simulink model "SpatialKineticsOffline"  (R2013a)
settings: Solver=ode4  StartTime=0.0  StopTime=tf  FixedStep=.001  RelTol=1e-3
PreLoadFcn:
  | load DarkLowerCoeffs
  | load DarkMiddleCoeffs
  | load DarkUpperCoeffs
  | load breaks
values from neighbouring files (symbols this model uses):
  alpha = [ -2.61*pcm -0.53*pcm ]    [SpatialKineticsOpenSourceMain.m]
  breaks = DarkLowerBreaks    [SpatialKineticsOpenSourceMain.m]
  BRIO = 4.266e7    (= 42660000)    [SpatialKineticsOpenSourceMain.m]
  cpc = 2414    [SpatialKineticsOpenSourceMain.m]
  cpp = 2414    [SpatialKineticsOpenSourceMain.m]
  DarkLowerCoeffs = ppDarkLower.coefs    [SpatialKineticsOpenSourceMain.m]
  DarkMiddleCoeffs = ppDarkMiddle.coefs    [SpatialKineticsOpenSourceMain.m]
  DarkRodWorthInserted = -5*Beta    (= -0.00815)    [SpatialKineticsOpenSourceMain.m]
  DarkUpperCoeffs = ppDarkUpper.coefs    [SpatialKineticsOpenSourceMain.m]
  downcomerTimeConstant = 5    [SpatialKineticsOpenSourceMain.m]
  downIO = 216.6*ones(1,3)    [SpatialKineticsOpenSourceMain.m]
  Kc1 = 1/(rho_secondary*V_secondary)    (= 0.00032726218348)    [SpatialKineticsOpenSourceMain.m]
  Kc2 = (h_secondary*A)/(cps*rho_secondary*V_secondary)    (= 1.23242359038)    [SpatialKineticsOpenSourceMain.m]
  Kh1 = 1/(rho_primary*V_primary)    (= 0.000447917898441)    [SpatialKineticsOpenSourceMain.m]
  Kh2 = (h_primary*A)/(cpp*rho_primary*V_primary)    (= 1.29038206968)    [SpatialKineticsOpenSourceMain.m]
  Kw1 = h_primary    (= 23800)    [SpatialKineticsOpenSourceMain.m]
  Kw2 = h_secondary    (= 24500)    [SpatialKineticsOpenSourceMain.m]
  Kw3 = A/(rho_tube*cpw*V_tube)    (= 0.000122049789882)    [SpatialKineticsOpenSourceMain.m]
  PHX_IO = [649.8 637.9 643.7]    [SpatialKineticsOpenSourceMain.m]
  PHX_PI_IO = 271.8    [SpatialKineticsOpenSourceMain.m]
  rate_pct = rate/100    [SpatialKineticsOfflineMain.m]
  rcp_activatetime = 20    [SpatialKineticsOpenSourceMain.m]
  rcpt = 0.1    [SpatialKineticsOpenSourceMain.m]
  reactor_PI_IO = 0.8574    [SpatialKineticsOpenSourceMain.m]
  SVIO = zeros(1,17)    [SpatialKineticsOpenSourceMain.m]
  Ts = 0.001    [SpatialKineticsOpenSourceMain.m]
  xfc0 = -Atemp\btemp*u0    [SpatialKineticsOpenSourceMain.m]
  zone1_IO = [1.041 0.01764 0.04848]    [SpatialKineticsOpenSourceMain.m]
  zone1_thermal_IO = [1044 658.3]    [SpatialKineticsOpenSourceMain.m]
  zone2_IO = [1.098 0.0186 0.05114]    [SpatialKineticsOpenSourceMain.m]
  zone2_thermal_IO = [1083 675.9]    [SpatialKineticsOpenSourceMain.m]
  zone3_IO = [0.9147 0.01549 0.04259]    [SpatialKineticsOpenSourceMain.m]
  zone3_thermal_IO = [1031 692.5]    [SpatialKineticsOpenSourceMain.m]
libraries: simulink x36
(part 4 of 5)

== system SpatialKineticsOffline/RX #3/Primary Heat Exchanger Lumped Model #5 ==
  Primary mass flow  in : Inport
  Primary temp in : Inport  Port=2
  Secondary temp in : Inport  Port=3
  Secondary mass flow in : Inport  Port=4
  Constant : Constant  Value=Kh1  SampleTime=Ts
  Constant1 : Constant  Value=Kh2  SampleTime=Ts
  Constant2 : Constant  Value=Kc1  SampleTime=Ts
  Constant3 : Constant  Value=Kc2  SampleTime=Ts
  Constant4 : Constant  Value=Kw1  SampleTime=Ts
  Constant5 : Constant  Value=Kw2  SampleTime=Ts
  Constant6 : Constant  Value=Kw3  SampleTime=Ts
  Constant7 : Constant  Value=cpp  SampleTime=Ts
  Demux : Demux  Outputs=3
  Display : Display
  Integrator : Integrator  InitialCondition=PHX_IO
  MATLAB Function : MATLAB Function  TreatAsAtomicUnit=on
  Mux2 : Mux  Inputs=7
  Product : Product
  Product1 : Product
  Sum : Sum  Inputs=|+-
  Terminator : Terminator
  W to MW : Gain  Gain=1e-6
  PHx1_Tho : Outport
  PHx1_Tco : Outport  Port=2
  PHx1_HXout : Outport  Port=3
  wires:
  Constant/1 -> Mux2/1
  Constant1/1 -> Mux2/2
  Constant2/1 -> Mux2/3
  Constant3/1 -> Mux2/4
  Constant4/1 -> Mux2/5
  Constant5/1 -> Mux2/6
  Constant6/1 -> Mux2/7
  Mux2/1 -> [PHXpar]
  MATLAB Function/1(dx) -> Integrator/1
  [PHXpar] -> MATLAB Function/6(hxpar)
  Primary temp in/1 -> [Thi], MATLAB Function/2(Thi_input)
  Secondary temp in/1 -> MATLAB Function/3(Tci_input)
  Secondary mass flow in/1 -> MATLAB Function/5(mdotc_input)
  Primary mass flow  in/1 -> [mdoth], MATLAB Function/4(mdoth_input)
  Demux/3 -> Terminator/1
  Demux/2 -> PHx1_Tco/1
  Demux/1 -> [Tho], PHx1_Tho/1
  Constant7/1 -> Product/2
  [mdoth] -> Product/1
  [Thi] -> Sum/1
  [Tho] -> Sum/2
  Product/1 -> Product1/1
  Sum/1 -> Product1/2
  Product1/1 -> W to MW/1
  W to MW/1 -> PHx1_HXout/1
  Integrator/1 -> Display/1, MATLAB Function/1(x), Demux/1

== system SpatialKineticsOffline/RX #3/Primary Heat Exchanger Lumped Model #6 ==
  Primary mass flow  in : Inport
  Primary temp in : Inport  Port=2
  Secondary temp in : Inport  Port=3
  Secondary mass flow in : Inport  Port=4
  Constant : Constant  Value=Kh1  SampleTime=Ts
  Constant1 : Constant  Value=Kh2  SampleTime=Ts
  Constant2 : Constant  Value=Kc1  SampleTime=Ts
  Constant3 : Constant  Value=Kc2  SampleTime=Ts
  Constant4 : Constant  Value=Kw1  SampleTime=Ts
  Constant5 : Constant  Value=Kw2  SampleTime=Ts
  Constant6 : Constant  Value=Kw3  SampleTime=Ts
  Constant7 : Constant  Value=cpp  SampleTime=Ts
  Demux : Demux  Outputs=3
  Display : Display
  Integrator : Integrator  InitialCondition=PHX_IO
  MATLAB Function : MATLAB Function  TreatAsAtomicUnit=on
  Mux2 : Mux  Inputs=7
  Product : Product
  Product1 : Product
  Sum : Sum  Inputs=|+-
  Terminator : Terminator
  W to MW : Gain  Gain=1e-6
  PHx1_Tho : Outport
  PHx1_Tco : Outport  Port=2
  PHx1_HXout : Outport  Port=3
  wires:
  Constant/1 -> Mux2/1
  Constant1/1 -> Mux2/2
  Constant2/1 -> Mux2/3
  Constant3/1 -> Mux2/4
  Constant4/1 -> Mux2/5
  Constant5/1 -> Mux2/6
  Constant6/1 -> Mux2/7
  Mux2/1 -> [PHXpar]
  MATLAB Function/1(dx) -> Integrator/1
  [PHXpar] -> MATLAB Function/6(hxpar)
  Primary temp in/1 -> [Thi], MATLAB Function/2(Thi_input)
  Secondary temp in/1 -> MATLAB Function/3(Tci_input)
  Secondary mass flow in/1 -> MATLAB Function/5(mdotc_input)
  Primary mass flow  in/1 -> [mdoth], MATLAB Function/4(mdoth_input)
  Integrator/1 -> Display/1, Demux/1, MATLAB Function/1(x)
  Demux/3 -> Terminator/1
  Demux/2 -> PHx1_Tco/1
  Demux/1 -> [Tho], PHx1_Tho/1
  Constant7/1 -> Product/2
  [mdoth] -> Product/1
  [Thi] -> Sum/1
  [Tho] -> Sum/2
  Product/1 -> Product1/1
  Sum/1 -> Product1/2
  Product1/1 -> W to MW/1
  W to MW/1 -> PHx1_HXout/1

== system SpatialKineticsOffline/RX #3/Ramp Power1 ==
  Max Demand : Inport
  Add : Sum
  Clock : Clock
  Ramp : simulink/Sources/Ramp  slope=rate_pct*42/60  start=tf/2  X0=-rate_pct*42/60*tf/2
  Ramp1 : simulink/Sources/Ramp  slope=-rate_pct*42/60  start=0  X0=0
  Switch : Switch  Threshold=tf/2
  Current Demand : Outport
  wires:
  Switch/1 -> Add/2
  Clock/1 -> Switch/2
  Ramp1/1 -> Switch/3
  Ramp/1 -> Switch/1
  Add/1 -> Current Demand/1
  Max Demand/1 -> Add/1

== system SpatialKineticsOffline/RX #3/Ramp Power2 ==
  Max Demand : Inport
  Add : Sum
  Clock : Clock
  Ramp : simulink/Sources/Ramp  slope=rate_pct*42/60  start=tf/2  X0=-rate_pct*42/60*tf/2
  Ramp1 : simulink/Sources/Ramp  slope=-rate_pct*42/60  start=0  X0=0
  Switch : Switch  Threshold=tf/2
  Current Demand : Outport
  wires:
  Switch/1 -> Add/2
  Clock/1 -> Switch/2
  Ramp1/1 -> Switch/3
  Ramp/1 -> Switch/1
  Add/1 -> Current Demand/1
  Max Demand/1 -> Add/1

== system SpatialKineticsOffline/RX #3/Ramp Power3 ==
  Max Demand : Inport
  Add : Sum
  Clock : Clock
  Ramp : simulink/Sources/Ramp  slope=rate_pct*42/60  start=tf/2  X0=-rate_pct*42/60*tf/2
  Ramp1 : simulink/Sources/Ramp  slope=-rate_pct*42/60  start=0  X0=0
  Switch : Switch  Threshold=tf/2
  Current Demand : Outport
  wires:
  Switch/1 -> Add/2
  Clock/1 -> Switch/2
  Ramp1/1 -> Switch/3
  Ramp/1 -> Switch/1
  Add/1 -> Current Demand/1
  Max Demand/1 -> Add/1

== system SpatialKineticsOffline/RX #3/Reactor Outlet Temperature PI Controller1 ==
  In1 : Inport
  Display : Display
  Display1 : Display
  Display2 : Display
  Gain2 : Gain  Gain=0.01
  Gain5 : Gain  Gain=100
  Integrator : Integrator  InitialCondition=reactor_PI_IO
  Kp : Gain  Gain=.01
  Saturation : Saturate  UpperLimit=1  LowerLimit=0
  Sum12 : Sum  Inputs=+-|
  Sum13 : Sum  Inputs=|+-
  Sum2 : Sum  Inputs=|++
  Out1 : Outport
  wires:
  In1/1 -> Kp/1, Sum13/1
  Sum2/1 -> Display/1, Sum12/1, Saturation/1
  Gain2/1 -> Integrator/1
  Integrator/1 -> Display2/1, Sum2/2
  Kp/1 -> Display1/1, Sum2/1
  Saturation/1 -> Sum12/2, Out1/1
  Sum12/1 -> Gain5/1
  Sum13/1 -> Gain2/1
  Gain5/1 -> Sum13/2

== system SpatialKineticsOffline/RX #3/Secondary-side RCP Dynamics #4 ==
  In1 : Inport
  Digital Clock #1 : DigitalClock  SampleTime=Ts
  RCP #1 : TransferFcn  Numerator=[rcpt]  Denominator=[1 rcpt]
  RCP Dynamics Switch #1 : Switch  Threshold=rcp_activatetime
  Out1 : Outport
  wires:
  In1/1 -> RCP #1/1, RCP Dynamics Switch #1/3
  Digital Clock #1/1 -> RCP Dynamics Switch #1/2
  RCP #1/1 -> RCP Dynamics Switch #1/1
  RCP Dynamics Switch #1/1 -> Out1/1

== system SpatialKineticsOffline/RX #3/Secondary-side RCP Dynamics #5 ==
  In1 : Inport
  Digital Clock#2 : DigitalClock  SampleTime=Ts
  RCP #2 : TransferFcn  Numerator=[rcpt]  Denominator=[1 rcpt]
  RCP Dynamics Switch #2 : Switch  Threshold=rcp_activatetime
  Out1 : Outport
  wires:
  RCP Dynamics Switch #2/1 -> Out1/1
  In1/1 -> RCP #2/1, RCP Dynamics Switch #2/3
  Digital Clock#2/1 -> RCP Dynamics Switch #2/2
  RCP #2/1 -> RCP Dynamics Switch #2/1

== system SpatialKineticsOffline/RX #3/Secondary-side RCP Dynamics #6 ==
  In1 : Inport
  Digital Clock #3 : DigitalClock  SampleTime=Ts
  RCP #3 : TransferFcn  Numerator=[rcpt]  Denominator=[1 rcpt]
  RCP Dynamics Switch #3 : Switch  Threshold=rcp_activatetime
  Out1 : Outport
  wires:
  RCP #3/1 -> RCP Dynamics Switch #3/1
  Digital Clock #3/1 -> RCP Dynamics Switch #3/2
  In1/1 -> RCP #3/1, RCP Dynamics Switch #3/3
  RCP Dynamics Switch #3/1 -> Out1/1

== system SpatialKineticsOffline/RX #4/Downcomer mixing dynamics ==
  PHX Primary Flow 1 : Inport
  PHX Primary Flow 2 : Inport  Port=2
  PHX Primary Flow 3 : Inport  Port=3
  PHX Primary Temp 1 : Inport  Port=4
  PHX Primary Temp 2 : Inport  Port=5
  PHX Primary Temp 3 : Inport  Port=6
  Constant5 : Constant  Value=[0,downcomerTimeConstant]
  Display : Display
  Integrator : Integrator  InitialCondition=downIO
  MATLAB Function1 : MATLAB Function  TreatAsAtomicUnit=on
  Primary Mass Flow Rate : Outport
  Temperature to Reactor T-H : Outport  Port=2
  wires:
  PHX Primary Flow 1/1 -> MATLAB Function1/1(m1)
  PHX Primary Flow 2/1 -> MATLAB Function1/2(m2)
  PHX Primary Flow 3/1 -> MATLAB Function1/3(m3)
  PHX Primary Temp 1/1 -> MATLAB Function1/4(t1)
  PHX Primary Temp 2/1 -> MATLAB Function1/5(t2)
  PHX Primary Temp 3/1 -> MATLAB Function1/6(t3)
  MATLAB Function1/3(xdot) -> Integrator/1
  Integrator/1 -> MATLAB Function1/8(x), Display/1
  MATLAB Function1/1(y) -> Temperature to Reactor T-H/1
  Constant5/1 -> MATLAB Function1/7(constants)
  MATLAB Function1/2(mtotal) -> Primary Mass Flow Rate/1

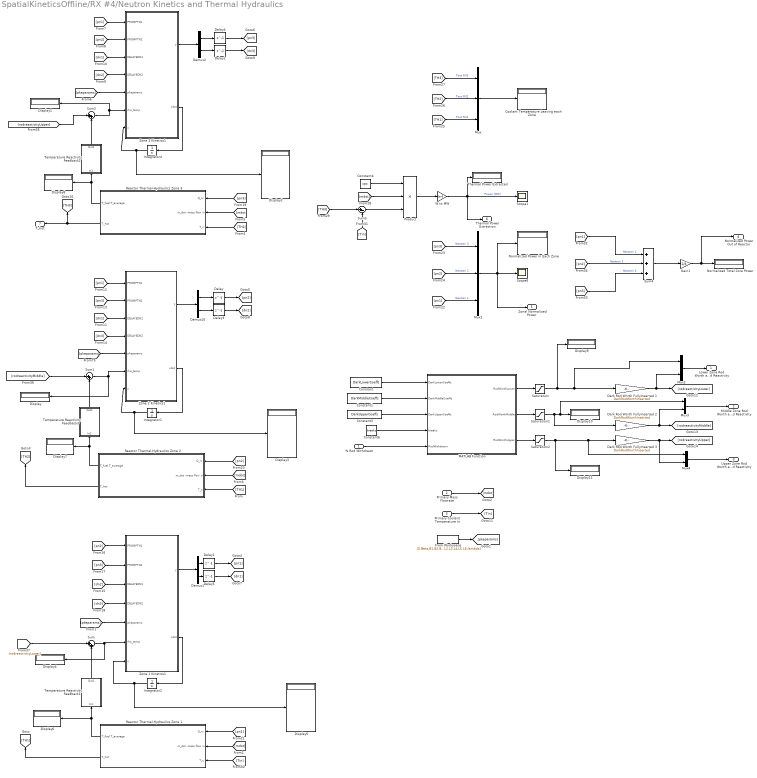
== system SpatialKineticsOffline/RX #4/Neutron Kinetics and Thermal Hydraulics ==
  % Rod Withdrawn : Inport
  Primary Mass Flowrate : Inport  Port=2
  Primary Coolant Temperature In : Inport  Port=3
  Constant : Constant  Value=DarkLowerCoeffs
  Constant1 : Constant  Value=DarkMiddleCoeffs
  Constant3 : Constant  Value=DarkUpperCoeffs
  Constant4 : Constant  Value=cpc
  Constant6 : Constant  Value=breaks
  Coolant Temperature Leaving each Zone : Display
  Dark Rod Worth FullyInserted 1 : Gain  Gain=DarkRodWorthInserted
  Dark Rod Worth FullyInserted 2 : Gain  Gain=DarkRodWorthInserted
  Dark Rod Worth FullyInserted 3 : Gain  Gain=DarkRodWorthInserted
  Delay{,1..5} (6 alike) : Delay  DelayLength=1  InitialCondition=0
  Demux1 : Demux  Outputs=2
  Demux10 : Demux  Outputs=2
  Demux2 : Demux  Outputs=2
  Display{,1..11} (12 alike) : Display
  From Workspace : FromWorkspace  VariableName=[0,Beta,B1,B2,B3,B4,B5,B6,L1,L2,L3,L4,L5,L6,lambda]  SampleTime=0
  Gain1 : Gain  Gain=1/3
  Integrator1 : Integrator  InitialCondition=zone2_IO
  Integrator2 : Integrator  InitialCondition=zone1_IO
  Integrator4 : Integrator  InitialCondition=zone3_IO
  MATLAB Function : MATLAB Function  TreatAsAtomicUnit=on
  Mux : Mux  Inputs=3
  Mux1 : Mux  Inputs=3
  Mux2 : Mux  Inputs=2
  Mux3 : Mux  Inputs=2
  Mux4 : Mux  Inputs=2
  Normalized Power in Each Zone : Display
  Normalized Total Core Power : Display
  Product : Product  Inputs=3
  Reactor Thermal-Hydraulics Zone 1 : Subsystem
  Reactor Thermal-Hydraulics Zone 2 : Subsystem
  Reactor Thermal-Hydraulics Zone 3 : Subsystem
  Saturation : Saturate  UpperLimit=inf  LowerLimit=0
  Saturation1 : Saturate  UpperLimit=inf  LowerLimit=0
  Saturation2 : Saturate  UpperLimit=inf  LowerLimit=0
  Scope1 : Scope
      settings: SaveName=ScopeData17
  Scope6 : Scope
      settings: SaveName=ScopeData16
  Sum : Sum  Inputs=|++
  Sum1 : Sum  Inputs=|++
  Sum2 : Sum  Inputs=|++
  Sum3 : Sum  Inputs=|+-
  Sum4 : Sum  Inputs=+++
  Temperature Reactivity Feedback1 : Subsystem
  Temperature Reactivity Feedback2 : Subsystem
  Temperature Reactivity Feedback3 : Subsystem
  Thermal Power Extracted : Display
  W to MW : Gain  Gain=1e-6
  Zone 1 Kinetics1 : MATLAB Function  TreatAsAtomicUnit=on
  Zone 2 Kinetics1 : MATLAB Function  TreatAsAtomicUnit=on
  Zone 3 Kinetics1 : MATLAB Function  TreatAsAtomicUnit=on
  Lower Zone Rod Worth and Reactivity : Outport
  Middle Zone Rod Worth and Reactivity : Outport  Port=2
  Upper Zone Rod Worth and Reactivity : Outport  Port=3
  Normalized Power Out of Reactor : Outport  Port=4
  Zonal Normalized Power : Outport  Port=5
  Thermal Power Extraction : Outport  Port=6
  T_hot : Outport  Port=7
  wires:
  [pkeparams] -> Zone 2 Kinetics1/5(pkeparams)
  Demux1/2 -> Delay5/1
  From Workspace/1 -> [pkeparams]
  Reactor Thermal-Hydraulics Zone 2/1(T_fuel,T_average) -> Display7/1, Temperature Reactivity Feedback3/1(In1)
  [TH1] -> Reactor Thermal-Hydraulics Zone 2/3(T_c)
  Temperature Reactivity Feedback3/1(Out1) -> Sum1/2
  [pkeparams] -> Zone 1 Kinetics1/5(pkeparams)
  Zone 1 Kinetics1/1(y) -> Demux1/1
  Reactor Thermal-Hydraulics Zone 1/1(T_fuel,T_average) -> Temperature Reactivity Feedback1/1(In1), Display6/1
  Temperature Reactivity Feedback1/1(Out1) -> Sum/2
  Demux1/1 -> Delay1/1
  Sum/1 -> Zone 1 Kinetics1/6(rho_temp), Display4/1
  [rodreactivityLower] -> Sum/1
  Sum1/1 -> Zone 2 Kinetics1/6(rho_temp), Display/1
  [rodreactivityMiddle] -> Sum1/1
  Mux/1 -> Coolant Temperature Leaving each Zone/1
  Reactor Thermal-Hydraulics Zone 1/2(T_hot) -> [TH1]
  [mdot] -> Reactor Thermal-Hydraulics Zone 2/2(m_dot -mass flow in)
  [mdot] -> Reactor Thermal-Hydraulics Zone 1/2(m_dot -mass flow in)
  Reactor Thermal-Hydraulics Zone 3/1(T_fuel,T_average) -> Display8/1, Temperature Reactivity Feedback2/1(In1)
  [TH2] -> Reactor Thermal-Hydraulics Zone 3/3(T_c)
  Reactor Thermal-Hydraulics Zone 3/2(T_hot) -> T_hot/1, [TH3]
  Temperature Reactivity Feedback2/1(Out1) -> Sum2/2
  Demux2/1 -> Delay4/1
  Sum2/1 -> Zone 3 Kinetics1/6(rho_temp), Display1/1
  [mdot] -> Reactor Thermal-Hydraulics Zone 3/2(m_dot -mass flow in)
  Delay5/1 -> [dn1]
  Demux2/2 -> Delay2/1
  Reactor Thermal-Hydraulics Zone 2/2(T_hot) -> [TH2]
  Demux10/1 -> Delay/1
  Demux10/2 -> Delay3/1
  Delay4/1 -> [pn3]
  Delay/1 -> [pn2]
  Delay1/1 -> [pn1]
  Delay3/1 -> [dn2]
  Delay2/1 -> [dn3]
  [rodreactivityUpper] -> Sum2/1
  [pn1] -> Zone 2 Kinetics1/1(PROMPTN1)
  [pn3] -> Zone 2 Kinetics1/2(PROMPTN2)
  [dn3] -> Zone 2 Kinetics1/4(DELAYEDN2)
  [dn1] -> Zone 2 Kinetics1/3(DELAYEDN1)
  [pn2] -> Zone 1 Kinetics1/1(PROMPTN1)
  [pn3] -> Zone 1 Kinetics1/2(PROMPTN2)
  [dn2] -> Zone 1 Kinetics1/3(DELAYEDN1)
  [dn3] -> Zone 1 Kinetics1/4(DELAYEDN2)
  [pn3] -> Reactor Thermal-Hydraulics Zone 3/1(Q_rx)
  [pn2] -> Reactor Thermal-Hydraulics Zone 2/1(Q_rx)
  [pn1] -> Reactor Thermal-Hydraulics Zone 1/1(Q_rx)
  Mux1/1 -> Scope6/1, Zonal Normalized Power/1, Normalized Power in Each Zone/1
  [pn1] -> Mux1/3  "Neutron 1"
  [pn3] -> Mux1/1  "Neutron 3"
  [pn2] -> Mux1/2  "Neutron 2"
  [TH1] -> Mux/3  "Tout RX1"
  [TH2] -> Mux/2  "Tout RX2"
  [TH3] -> Mux/1  "Tout RX3"
  Constant4/1 -> Product/1
  [mdot] -> Product/2
  Sum3/1 -> Product/3
  [TH3] -> Sum3/1
  [Tin] -> Reactor Thermal-Hydraulics Zone 1/3(T_c)
  [Tin] -> Sum3/2
  Product/1 -> W to MW/1
  W to MW/1 -> Scope1/1, Thermal Power Extraction/1, Thermal Power Extracted/1  "Power (MW)"
  [pn1] -> Sum4/1  "Neutron 1"
  [pn3] -> Sum4/3  "Neutron 3"
  [pn2] -> Sum4/2  "Neutron 2"
  Sum4/1 -> Gain1/1
  Gain1/1 -> Normalized Power Out of Reactor/1, Normalized Total Core Power/1
  Constant6/1 -> MATLAB Function/4(breaks)
  Constant3/1 -> MATLAB Function/3(DarkUpperCoeffs)
  Constant1/1 -> MATLAB Function/2(DarkMiddleCoeffs)
  Constant/1 -> MATLAB Function/1(DarkLowerCoeffs)
  MATLAB Function/1(RodWorthLower) -> Saturation/1
  MATLAB Function/2(RodWorthMiddle) -> Saturation1/1
  MATLAB Function/3(RodWorthUpper) -> Saturation2/1
  % Rod Withdrawn/1 -> MATLAB Function/5(RodWithdrawn)
  Saturation/1 -> Mux2/1, Dark Rod Worth FullyInserted 1/1, Display9/1
  Saturation1/1 -> Dark Rod Worth FullyInserted 2/1, Mux3/1, Display10/1
  Saturation2/1 -> Mux4/1, Dark Rod Worth FullyInserted 3/1, Display11/1
  Dark Rod Worth FullyInserted 1/1 -> Mux2/2, [rodreactivityLower]
  Dark Rod Worth FullyInserted 2/1 -> Mux3/2, [rodreactivityMiddle]
  Dark Rod Worth FullyInserted 3/1 -> Mux4/2, [rodreactivityUpper]
  Primary Mass Flowrate/1 -> [mdot]
  Primary Coolant Temperature In/1 -> [Tin]
  Mux2/1 -> Lower Zone Rod Worth and Reactivity/1
  Mux3/1 -> Middle Zone Rod Worth and Reactivity/1
  Mux4/1 -> Upper Zone Rod Worth and Reactivity/1
  Integrator4/1 -> Display2/1, Zone 3 Kinetics1/7(x)
  Zone 3 Kinetics1/2(xdot) -> Integrator4/1
  [pkeparams] -> Zone 3 Kinetics1/5(pkeparams)
  [dn2] -> Zone 3 Kinetics1/4(DELAYEDN2)
  [dn1] -> Zone 3 Kinetics1/3(DELAYEDN1)
  [pn2] -> Zone 3 Kinetics1/2(PROMPTN2)
  [pn1] -> Zone 3 Kinetics1/1(PROMPTN1)
  Zone 3 Kinetics1/1(y) -> Demux2/1
  Zone 2 Kinetics1/2(xdot) -> Integrator1/1
  Integrator1/1 -> Display3/1, Zone 2 Kinetics1/7(x)
  Zone 2 Kinetics1/1(y) -> Demux10/1
  Zone 1 Kinetics1/2(xdot) -> Integrator2/1
  Integrator2/1 -> Display5/1, Zone 1 Kinetics1/7(x)

== system SpatialKineticsOffline/RX #4/PI Controller with Integral Anti-windup for HX4 ==
  HX Power Produced : Inport
  Power Setpoint : Inport  Port=2
  Cold_flow_high5 : Constant  Value=370
  Cold_flow_low2 : Constant  Value=0
  Display : Display
  Gain5 : Gain  Gain=15
  Integrator2 : Integrator  InitialCondition=PHX_PI_IO
  Ki2 : Gain  Gain=0.14145998
  Kp2 : Gain  Gain=1.083074
  Saturation Dynamic2 : simulink/Discontinuities/Saturation Dynamic  OutMin=[]  OutMax=[]  OutDataTypeStr=Inherit: Same as second input  OutDataType=fixdt(1, 16)  OutScaling=2^-10  DoSatur=off
  Sum12 : Sum  Inputs=+-|
  Sum13 : Sum  Inputs=|+-
  Sum14 : Sum  Inputs=|+-
  Sum15 : Sum  Inputs=|++
  Control Action : Outport
  wires:
  HX Power Produced/1 -> Sum14/2
  Cold_flow_low2/1 -> Saturation Dynamic2/3
  Cold_flow_high5/1 -> Saturation Dynamic2/1
  Sum14/1 -> Kp2/1, Sum13/1
  Power Setpoint/1 -> Sum14/1
  Sum12/1 -> Gain5/1
  Gain5/1 -> Sum13/2
  Sum13/1 -> Ki2/1
  Ki2/1 -> Integrator2/1
  Kp2/1 -> Sum15/1
  Saturation Dynamic2/1 -> Control Action/1, Sum12/2
  Sum15/1 -> Saturation Dynamic2/2, Sum12/1
  Integrator2/1 -> Display/1, Sum15/2

== system SpatialKineticsOffline/RX #4/PI Controller with Integral Anti-windup for HX5 ==
  HX Power Produced : Inport
  Power Setpoint : Inport  Port=2
  Cold_flow_high5 : Constant  Value=370
  Cold_flow_low2 : Constant  Value=0
  Display : Display
  Gain5 : Gain  Gain=15
  Integrator2 : Integrator  InitialCondition=PHX_PI_IO
  Ki2 : Gain  Gain=0.14145998
  Kp2 : Gain  Gain=1.083074
  Saturation Dynamic2 : simulink/Discontinuities/Saturation Dynamic  OutMin=[]  OutMax=[]  OutDataTypeStr=Inherit: Same as second input  OutDataType=fixdt(1, 16)  OutScaling=2^-10  DoSatur=off
  Sum12 : Sum  Inputs=+-|
  Sum13 : Sum  Inputs=|+-
  Sum14 : Sum  Inputs=|+-
  Sum15 : Sum  Inputs=|++
  Control Action : Outport
  wires:
  HX Power Produced/1 -> Sum14/2
  Cold_flow_low2/1 -> Saturation Dynamic2/3
  Cold_flow_high5/1 -> Saturation Dynamic2/1
  Sum14/1 -> Kp2/1, Sum13/1
  Power Setpoint/1 -> Sum14/1
  Sum12/1 -> Gain5/1
  Integrator2/1 -> Display/1, Sum15/2
  Gain5/1 -> Sum13/2
  Sum13/1 -> Ki2/1
  Ki2/1 -> Integrator2/1
  Kp2/1 -> Sum15/1
  Saturation Dynamic2/1 -> Control Action/1, Sum12/2
  Sum15/1 -> Saturation Dynamic2/2, Sum12/1

== system SpatialKineticsOffline/RX #4/PI Controller with Integral Anti-windup for HX6 ==
  HX Power Produced : Inport
  Power Setpoint : Inport  Port=2
  Cold_flow_high5 : Constant  Value=370
  Cold_flow_low2 : Constant  Value=0
  Display : Display
  Gain5 : Gain  Gain=15
  Integrator2 : Integrator  InitialCondition=PHX_PI_IO
  Ki2 : Gain  Gain=0.14145998
  Kp2 : Gain  Gain=1.083074
  Saturation Dynamic2 : simulink/Discontinuities/Saturation Dynamic  OutMin=[]  OutMax=[]  OutDataTypeStr=Inherit: Same as second input  OutDataType=fixdt(1, 16)  OutScaling=2^-10  DoSatur=off
  Sum12 : Sum  Inputs=+-|
  Sum13 : Sum  Inputs=|+-
  Sum14 : Sum  Inputs=|+-
  Sum15 : Sum  Inputs=|++
  Control Action : Outport
  wires:
  HX Power Produced/1 -> Sum14/2
  Cold_flow_low2/1 -> Saturation Dynamic2/3
  Cold_flow_high5/1 -> Saturation Dynamic2/1
  Sum14/1 -> Kp2/1, Sum13/1
  Power Setpoint/1 -> Sum14/1
  Sum12/1 -> Gain5/1
  Integrator2/1 -> Display/1, Sum15/2
  Gain5/1 -> Sum13/2
  Sum13/1 -> Ki2/1
  Ki2/1 -> Integrator2/1
  Kp2/1 -> Sum15/1
  Saturation Dynamic2/1 -> Control Action/1, Sum12/2
  Sum15/1 -> Saturation Dynamic2/2, Sum12/1

== system SpatialKineticsOffline/RX #4/Parasitic Heat Loss Resulting from DRACS HXs2 ==
  "T_hot " : Inport
  T_cold : Inport  Port=2
  Primary Mass Flow Rate : Inport  Port=3
  MATLAB Function : MATLAB Function  TreatAsAtomicUnit=on
  Specific heat capacity of primary coolant : Constant  Value=cpp
  Total Power Out : Outport
  Power Lost : Outport  Port=2
  Hot Leg Reduction : Outport  Port=3
  wires:
  MATLAB Function/3(Th_red) -> Hot Leg Reduction/1
  MATLAB Function/2(Ploss_MW) -> Power Lost/1
  MATLAB Function/1(P_MW) -> Total Power Out/1
  "T_hot "/1 -> MATLAB Function/1(T_hot)
  T_cold/1 -> MATLAB Function/2(T_cold)
  Primary Mass Flow Rate/1 -> MATLAB Function/3(mdoth)
  Specific heat capacity of primary coolant/1 -> MATLAB Function/4(cpp)

== system SpatialKineticsOffline/RX #4/Primary Heat Exchanger Lumped Model #4 ==
  Primary mass flow  in : Inport
  Primary temp in : Inport  Port=2
  Secondary temp in : Inport  Port=3
  Secondary mass flow in : Inport  Port=4
  Constant : Constant  Value=Kh1  SampleTime=Ts
  Constant1 : Constant  Value=Kh2  SampleTime=Ts
  Constant2 : Constant  Value=Kc1  SampleTime=Ts
  Constant3 : Constant  Value=Kc2  SampleTime=Ts
  Constant4 : Constant  Value=Kw1  SampleTime=Ts
  Constant5 : Constant  Value=Kw2  SampleTime=Ts
  Constant6 : Constant  Value=Kw3  SampleTime=Ts
  Constant7 : Constant  Value=cpp  SampleTime=Ts
  Demux : Demux  Outputs=3
  Display : Display
  Integrator : Integrator  InitialCondition=PHX_IO
  MATLAB Function : MATLAB Function  TreatAsAtomicUnit=on
  Mux2 : Mux  Inputs=7
  Product : Product
  Product1 : Product
  Sum : Sum  Inputs=|+-
  Terminator : Terminator
  W to MW : Gain  Gain=1e-6
  PHx1_Tho : Outport
  PHx1_Tco : Outport  Port=2
  PHx1_HXout : Outport  Port=3
  wires:
  Constant/1 -> Mux2/1
  Constant1/1 -> Mux2/2
  Constant2/1 -> Mux2/3
  Constant3/1 -> Mux2/4
  Constant4/1 -> Mux2/5
  Constant5/1 -> Mux2/6
  Constant6/1 -> Mux2/7
  Mux2/1 -> [PHXpar]
  MATLAB Function/1(dx) -> Integrator/1
  [PHXpar] -> MATLAB Function/6(hxpar)
  Primary temp in/1 -> [Thi], MATLAB Function/2(Thi_input)
  Secondary temp in/1 -> MATLAB Function/3(Tci_input)
  Secondary mass flow in/1 -> MATLAB Function/5(mdotc_input)
  Primary mass flow  in/1 -> [mdoth], MATLAB Function/4(mdoth_input)
  Integrator/1 -> Display/1, Demux/1, MATLAB Function/1(x)
  Demux/3 -> Terminator/1
  Demux/2 -> PHx1_Tco/1
  Demux/1 -> [Tho], PHx1_Tho/1
  Constant7/1 -> Product/2
  [mdoth] -> Product/1
  [Thi] -> Sum/1
  [Tho] -> Sum/2
  Product/1 -> Product1/1
  Sum/1 -> Product1/2
  Product1/1 -> W to MW/1
  W to MW/1 -> PHx1_HXout/1

== system SpatialKineticsOffline/RX #4/Primary Heat Exchanger Lumped Model #5 ==
  Primary mass flow  in : Inport
  Primary temp in : Inport  Port=2
  Secondary temp in : Inport  Port=3
  Secondary mass flow in : Inport  Port=4
  Constant : Constant  Value=Kh1  SampleTime=Ts
  Constant1 : Constant  Value=Kh2  SampleTime=Ts
  Constant2 : Constant  Value=Kc1  SampleTime=Ts
  Constant3 : Constant  Value=Kc2  SampleTime=Ts
  Constant4 : Constant  Value=Kw1  SampleTime=Ts
  Constant5 : Constant  Value=Kw2  SampleTime=Ts
  Constant6 : Constant  Value=Kw3  SampleTime=Ts
  Constant7 : Constant  Value=cpp  SampleTime=Ts
  Demux : Demux  Outputs=3
  Display : Display
  Integrator : Integrator  InitialCondition=PHX_IO
  MATLAB Function : MATLAB Function  TreatAsAtomicUnit=on
  Mux2 : Mux  Inputs=7
  Product : Product
  Product1 : Product
  Sum : Sum  Inputs=|+-
  Terminator : Terminator
  W to MW : Gain  Gain=1e-6
  PHx1_Tho : Outport
  PHx1_Tco : Outport  Port=2
  PHx1_HXout : Outport  Port=3
  wires:
  Constant/1 -> Mux2/1
  Constant1/1 -> Mux2/2
  Constant2/1 -> Mux2/3
  Constant3/1 -> Mux2/4
  Constant4/1 -> Mux2/5
  Constant5/1 -> Mux2/6
  Constant6/1 -> Mux2/7
  Mux2/1 -> [PHXpar]
  MATLAB Function/1(dx) -> Integrator/1
  [PHXpar] -> MATLAB Function/6(hxpar)
  Primary temp in/1 -> MATLAB Function/2(Thi_input), [Thi]
  Secondary temp in/1 -> MATLAB Function/3(Tci_input)
  Secondary mass flow in/1 -> MATLAB Function/5(mdotc_input)
  Primary mass flow  in/1 -> [mdoth], MATLAB Function/4(mdoth_input)
  Integrator/1 -> Display/1, Demux/1, MATLAB Function/1(x)
  Demux/3 -> Terminator/1
  Demux/2 -> PHx1_Tco/1
  Demux/1 -> [Tho], PHx1_Tho/1
  Constant7/1 -> Product/2
  [mdoth] -> Product/1
  [Thi] -> Sum/1
  [Tho] -> Sum/2
  Product/1 -> Product1/1
  Sum/1 -> Product1/2
  Product1/1 -> W to MW/1
  W to MW/1 -> PHx1_HXout/1

== system SpatialKineticsOffline/RX #4/Primary Heat Exchanger Lumped Model #6 ==
  Primary mass flow  in : Inport
  Primary temp in : Inport  Port=2
  Secondary temp in : Inport  Port=3
  Secondary mass flow in : Inport  Port=4
  Constant : Constant  Value=Kh1  SampleTime=Ts
  Constant1 : Constant  Value=Kh2  SampleTime=Ts
  Constant2 : Constant  Value=Kc1  SampleTime=Ts
  Constant3 : Constant  Value=Kc2  SampleTime=Ts
  Constant4 : Constant  Value=Kw1  SampleTime=Ts
  Constant5 : Constant  Value=Kw2  SampleTime=Ts
  Constant6 : Constant  Value=Kw3  SampleTime=Ts
  Constant7 : Constant  Value=cpp  SampleTime=Ts
  Demux : Demux  Outputs=3
  Display : Display
  Integrator : Integrator  InitialCondition=PHX_IO
  MATLAB Function : MATLAB Function  TreatAsAtomicUnit=on
  Mux2 : Mux  Inputs=7
  Product : Product
  Product1 : Product
  Sum : Sum  Inputs=|+-
  Terminator : Terminator
  W to MW : Gain  Gain=1e-6
  PHx1_Tho : Outport
  PHx1_Tco : Outport  Port=2
  PHx1_HXout : Outport  Port=3
  wires:
  Constant/1 -> Mux2/1
  Constant1/1 -> Mux2/2
  Constant2/1 -> Mux2/3
  Constant3/1 -> Mux2/4
  Constant4/1 -> Mux2/5
  Constant5/1 -> Mux2/6
  Constant6/1 -> Mux2/7
  Mux2/1 -> [PHXpar]
  MATLAB Function/1(dx) -> Integrator/1
  [PHXpar] -> MATLAB Function/6(hxpar)
  Primary temp in/1 -> [Thi], MATLAB Function/2(Thi_input)
  Secondary temp in/1 -> MATLAB Function/3(Tci_input)
  Secondary mass flow in/1 -> MATLAB Function/5(mdotc_input)
  Primary mass flow  in/1 -> [mdoth], MATLAB Function/4(mdoth_input)
  Integrator/1 -> Display/1, Demux/1, MATLAB Function/1(x)
  Demux/3 -> Terminator/1
  Demux/2 -> PHx1_Tco/1
  Demux/1 -> [Tho], PHx1_Tho/1
  Constant7/1 -> Product/2
  [mdoth] -> Product/1
  [Thi] -> Sum/1
  [Tho] -> Sum/2
  Product/1 -> Product1/1
  Sum/1 -> Product1/2
  Product1/1 -> W to MW/1
  W to MW/1 -> PHx1_HXout/1

== system SpatialKineticsOffline/RX #4/Ramp Power1 ==
  Max Demand : Inport
  Add : Sum
  Clock : Clock
  Ramp : simulink/Sources/Ramp  slope=rate_pct*42/60  start=tf/2  X0=-rate_pct*42/60*tf/2
  Ramp1 : simulink/Sources/Ramp  slope=-rate_pct*42/60  start=0  X0=0
  Switch : Switch  Threshold=tf/2
  Current Demand : Outport
  wires:
  Switch/1 -> Add/2
  Clock/1 -> Switch/2
  Ramp1/1 -> Switch/3
  Ramp/1 -> Switch/1
  Add/1 -> Current Demand/1
  Max Demand/1 -> Add/1

== system SpatialKineticsOffline/RX #4/Ramp Power2 ==
  Max Demand : Inport
  Add : Sum
  Clock : Clock
  Ramp : simulink/Sources/Ramp  slope=rate_pct*42/60  start=tf/2  X0=-rate_pct*42/60*tf/2
  Ramp1 : simulink/Sources/Ramp  slope=-rate_pct*42/60  start=0  X0=0
  Switch : Switch  Threshold=tf/2
  Current Demand : Outport
  wires:
  Switch/1 -> Add/2
  Clock/1 -> Switch/2
  Ramp1/1 -> Switch/3
  Ramp/1 -> Switch/1
  Add/1 -> Current Demand/1
  Max Demand/1 -> Add/1

== system SpatialKineticsOffline/RX #4/Ramp Power3 ==
  Max Demand : Inport
  Add : Sum
  Clock : Clock
  Ramp : simulink/Sources/Ramp  slope=rate_pct*42/60  start=tf/2  X0=-rate_pct*42/60*tf/2
  Ramp1 : simulink/Sources/Ramp  slope=-rate_pct*42/60  start=0  X0=0
  Switch : Switch  Threshold=tf/2
  Current Demand : Outport
  wires:
  Switch/1 -> Add/2
  Clock/1 -> Switch/2
  Ramp1/1 -> Switch/3
  Ramp/1 -> Switch/1
  Add/1 -> Current Demand/1
  Max Demand/1 -> Add/1

== system SpatialKineticsOffline/RX #4/Reactor Outlet Temperature PI Controller1 ==
  In1 : Inport
  Display : Display
  Display1 : Display
  Display2 : Display
  Gain2 : Gain  Gain=0.01
  Gain5 : Gain  Gain=100
  Integrator : Integrator  InitialCondition=reactor_PI_IO
  Kp : Gain  Gain=.01
  Saturation : Saturate  UpperLimit=1  LowerLimit=0
  Sum12 : Sum  Inputs=+-|
  Sum13 : Sum  Inputs=|+-
  Sum2 : Sum  Inputs=|++
  Out1 : Outport
  wires:
  In1/1 -> Kp/1, Sum13/1
  Sum2/1 -> Display/1, Sum12/1, Saturation/1
  Gain2/1 -> Integrator/1
  Integrator/1 -> Display2/1, Sum2/2
  Kp/1 -> Display1/1, Sum2/1
  Saturation/1 -> Sum12/2, Out1/1
  Sum12/1 -> Gain5/1
  Sum13/1 -> Gain2/1
  Gain5/1 -> Sum13/2

== system SpatialKineticsOffline/RX #4/Secondary-side RCP Dynamics #4 ==
  In1 : Inport
  Digital Clock #1 : DigitalClock  SampleTime=Ts
  RCP #1 : TransferFcn  Numerator=[rcpt]  Denominator=[1 rcpt]
  RCP Dynamics Switch #1 : Switch  Threshold=rcp_activatetime
  Out1 : Outport
  wires:
  In1/1 -> RCP #1/1, RCP Dynamics Switch #1/3
  Digital Clock #1/1 -> RCP Dynamics Switch #1/2
  RCP #1/1 -> RCP Dynamics Switch #1/1
  RCP Dynamics Switch #1/1 -> Out1/1

== system SpatialKineticsOffline/RX #4/Secondary-side RCP Dynamics #5 ==
  In1 : Inport
  Digital Clock#2 : DigitalClock  SampleTime=Ts
  RCP #2 : TransferFcn  Numerator=[rcpt]  Denominator=[1 rcpt]
  RCP Dynamics Switch #2 : Switch  Threshold=rcp_activatetime
  Out1 : Outport
  wires:
  RCP Dynamics Switch #2/1 -> Out1/1
  In1/1 -> RCP #2/1, RCP Dynamics Switch #2/3
  Digital Clock#2/1 -> RCP Dynamics Switch #2/2
  RCP #2/1 -> RCP Dynamics Switch #2/1

== system SpatialKineticsOffline/RX #4/Secondary-side RCP Dynamics #6 ==
  In1 : Inport
  Digital Clock #3 : DigitalClock  SampleTime=Ts
  RCP #3 : TransferFcn  Numerator=[rcpt]  Denominator=[1 rcpt]
  RCP Dynamics Switch #3 : Switch  Threshold=rcp_activatetime
  Out1 : Outport
  wires:
  RCP #3/1 -> RCP Dynamics Switch #3/1
  Digital Clock #3/1 -> RCP Dynamics Switch #3/2
  In1/1 -> RCP #3/1, RCP Dynamics Switch #3/3
  RCP Dynamics Switch #3/1 -> Out1/1

== system SpatialKineticsOffline/RX #1/Neutron Kinetics and Thermal Hydraulics/Reactor Thermal-Hydraulics Zone 1 ==
  Q_rx : Inport
  m_dot -mass flow in : Inport  Port=2
  T_c : Inport  Port=3
  Demux : Demux  Outputs=3
  Display : Display
  From Workspace : FromWorkspace  VariableName=[0,cpc,cpf,mc,mf,uh,Ar]  SampleTime=0
  Integrator : Integrator  InitialCondition=zone1_thermal_IO
  MATLAB Function : MATLAB Function  TreatAsAtomicUnit=on
  Mux : Mux  Inputs=2
  T_fuel,T_average : Outport
  T_hot : Outport  Port=2
  wires:
  MATLAB Function/2(x_dot) -> Integrator/1
  Integrator/1 -> Display/1, MATLAB Function/5(x)
  m_dot -mass flow in/1 -> MATLAB Function/1(m_dot)
  Demux/2 -> Mux/2
  T_c/1 -> MATLAB Function/4(T_c)
  From Workspace/1 -> MATLAB Function/3(constants)
  Q_rx/1 -> MATLAB Function/2(Q_rx)
  MATLAB Function/1(y) -> Demux/1
  Demux/1 -> Mux/1  "T_fuel"
  Mux/1 -> T_fuel,T_average/1
  Demux/3 -> T_hot/1

== system SpatialKineticsOffline/RX #1/Neutron Kinetics and Thermal Hydraulics/Reactor Thermal-Hydraulics Zone 2 ==
  Q_rx : Inport
  m_dot -mass flow in : Inport  Port=2
  T_c : Inport  Port=3
  Demux : Demux  Outputs=3
  Display : Display
  From Workspace : FromWorkspace  VariableName=[0,cpc,cpf,mc,mf,uh,Ar]  SampleTime=0
  Integrator1 : Integrator  InitialCondition=zone2_thermal_IO
  MATLAB Function : MATLAB Function  TreatAsAtomicUnit=on
  Mux : Mux  Inputs=2
  Scope : Scope
      settings: SaveName=ScopeData8
  Scope1 : Scope
      settings: SaveName=ScopeData9
  Scope2 : Scope
      settings: SaveName=ScopeData2
  T_fuel,T_average : Outport
  T_hot : Outport  Port=2
  wires:
  MATLAB Function/2(x_dot) -> Integrator1/1
  Integrator1/1 -> Display/1, MATLAB Function/5(x)
  m_dot -mass flow in/1 -> MATLAB Function/1(m_dot)
  Demux/2 -> Scope1/1, Mux/2  "T_average"
  T_c/1 -> MATLAB Function/4(T_c)
  From Workspace/1 -> MATLAB Function/3(constants)
  Q_rx/1 -> MATLAB Function/2(Q_rx)
  MATLAB Function/1(y) -> Demux/1
  Demux/1 -> Mux/1  "T_fuel"
  Mux/1 -> Scope2/1, T_fuel,T_average/1
  Demux/3 -> T_hot/1, Scope/1  "T_hot"

== system SpatialKineticsOffline/RX #1/Neutron Kinetics and Thermal Hydraulics/Reactor Thermal-Hydraulics Zone 3 ==
  Q_rx : Inport
  m_dot -mass flow in : Inport  Port=2
  T_c : Inport  Port=3
  Demux : Demux  Outputs=3
  Display : Display
  From Workspace : FromWorkspace  VariableName=[0,cpc,cpf,mc,mf,uh,Ar]  SampleTime=0
  Integrator1 : Integrator  InitialCondition=zone3_thermal_IO
  MATLAB Function : MATLAB Function  TreatAsAtomicUnit=on
  Mux : Mux  Inputs=2
  T_fuel,T_average : Outport
  T_hot : Outport  Port=2
  wires:
  MATLAB Function/2(x_dot) -> Integrator1/1
  Integrator1/1 -> MATLAB Function/5(x), Display/1
  m_dot -mass flow in/1 -> MATLAB Function/1(m_dot)
  Demux/2 -> Mux/2
  T_c/1 -> MATLAB Function/4(T_c)
  From Workspace/1 -> MATLAB Function/3(constants)
  Q_rx/1 -> MATLAB Function/2(Q_rx)
  MATLAB Function/1(y) -> Demux/1
  Demux/1 -> Mux/1  "T_fuel"
  Mux/1 -> T_fuel,T_average/1
  Demux/3 -> T_hot/1

== system SpatialKineticsOffline/RX #1/Neutron Kinetics and Thermal Hydraulics/Temperature Reactivity Feedback ==
  In1 : Inport
  Sum : Sum  Inputs=|+-
  reactivity feedback matrix : Gain  Gain=alpha  Multiplication=Matrix(K*u)
  reactivity reference temperature : Constant  Value=xfc0  VectorParams1D=off
  Out1 : Outport
  wires:
  reactivity reference temperature/1 -> Sum/2
  Sum/1 -> reactivity feedback matrix/1
  reactivity feedback matrix/1 -> Out1/1
  In1/1 -> Sum/1

== system SpatialKineticsOffline/RX #1/Neutron Kinetics and Thermal Hydraulics/Temperature Reactivity Feedback2 ==
  In1 : Inport
  Sum : Sum  Inputs=|+-
  reactivity feedback matrix : Gain  Gain=alpha  Multiplication=Matrix(K*u)
  reactivity reference temperature : Constant  Value=xfc0  VectorParams1D=off
  Out1 : Outport
  wires:
  reactivity reference temperature/1 -> Sum/2
  Sum/1 -> reactivity feedback matrix/1
  reactivity feedback matrix/1 -> Out1/1
  In1/1 -> Sum/1

== system SpatialKineticsOffline/RX #1/Neutron Kinetics and Thermal Hydraulics/Temperature Reactivity Feedback3 ==
  In1 : Inport
  Sum : Sum  Inputs=|+-
  reactivity feedback matrix : Gain  Gain=alpha  Multiplication=Matrix(K*u)
  reactivity reference temperature : Constant  Value=xfc0  VectorParams1D=off
  Out1 : Outport
  wires:
  reactivity reference temperature/1 -> Sum/2
  Sum/1 -> reactivity feedback matrix/1
  reactivity feedback matrix/1 -> Out1/1
  In1/1 -> Sum/1

== system SpatialKineticsOffline/RX #2/Neutron Kinetics and Thermal Hydraulics1/Reactor Thermal-Hydraulics Zone 1 ==
  Q_rx : Inport
  m_dot -mass flow in : Inport  Port=2
  T_c : Inport  Port=3
  Demux : Demux  Outputs=3
  Display : Display
  From Workspace : FromWorkspace  VariableName=[0,cpc,cpf,mc,mf,uh,Ar]  SampleTime=0
  Integrator1 : Integrator  InitialCondition=zone1_thermal_IO
  MATLAB Function : MATLAB Function  TreatAsAtomicUnit=on
  Mux : Mux  Inputs=2
  Scope : Scope
      settings: SaveName=ScopeData8
  Scope1 : Scope
      settings: SaveName=ScopeData9
  Scope2 : Scope
      settings: SaveName=ScopeData2
  T_fuel,T_average : Outport
  T_hot : Outport  Port=2
  wires:
  MATLAB Function/2(x_dot) -> Integrator1/1
  Integrator1/1 -> Display/1, MATLAB Function/5(x)
  m_dot -mass flow in/1 -> MATLAB Function/1(m_dot)
  Demux/2 -> Scope1/1, Mux/2  "T_average"
  T_c/1 -> MATLAB Function/4(T_c)
  From Workspace/1 -> MATLAB Function/3(constants)
  Q_rx/1 -> MATLAB Function/2(Q_rx)
  MATLAB Function/1(y) -> Demux/1
  Demux/1 -> Mux/1  "T_fuel"
  Mux/1 -> Scope2/1, T_fuel,T_average/1
  Demux/3 -> T_hot/1, Scope/1  "T_hot"

== system SpatialKineticsOffline/RX #2/Neutron Kinetics and Thermal Hydraulics1/Reactor Thermal-Hydraulics Zone 2 ==
  Q_rx : Inport
  m_dot -mass flow in : Inport  Port=2
  T_c : Inport  Port=3
  Demux : Demux  Outputs=3
  Display : Display
  From Workspace : FromWorkspace  VariableName=[0,cpc,cpf,mc,mf,uh,Ar]  SampleTime=0
  Integrator1 : Integrator  InitialCondition=zone2_thermal_IO
  MATLAB Function : MATLAB Function  TreatAsAtomicUnit=on
  Mux : Mux  Inputs=2
  Scope : Scope
      settings: SaveName=ScopeData8
  Scope1 : Scope
      settings: SaveName=ScopeData9
  Scope2 : Scope
      settings: SaveName=ScopeData2
  T_fuel,T_average : Outport
  T_hot : Outport  Port=2
  wires:
  MATLAB Function/2(x_dot) -> Integrator1/1
  Integrator1/1 -> Display/1, MATLAB Function/5(x)
  m_dot -mass flow in/1 -> MATLAB Function/1(m_dot)
  Demux/2 -> Scope1/1, Mux/2  "T_average"
  T_c/1 -> MATLAB Function/4(T_c)
  From Workspace/1 -> MATLAB Function/3(constants)
  Q_rx/1 -> MATLAB Function/2(Q_rx)
  MATLAB Function/1(y) -> Demux/1
  Demux/1 -> Mux/1  "T_fuel"
  Mux/1 -> Scope2/1, T_fuel,T_average/1
  Demux/3 -> T_hot/1, Scope/1  "T_hot"

== system SpatialKineticsOffline/RX #2/Neutron Kinetics and Thermal Hydraulics1/Reactor Thermal-Hydraulics Zone 3 ==
  Q_rx : Inport
  m_dot -mass flow in : Inport  Port=2
  T_c : Inport  Port=3
  Demux : Demux  Outputs=3
  Display : Display
  From Workspace : FromWorkspace  VariableName=[0,cpc,cpf,mc,mf,uh,Ar]  SampleTime=0
  Integrator1 : Integrator  InitialCondition=zone3_thermal_IO
  MATLAB Function : MATLAB Function  TreatAsAtomicUnit=on
  Mux : Mux  Inputs=2
  Scope : Scope
      settings: SaveName=ScopeData8
  Scope1 : Scope
      settings: SaveName=ScopeData9
  Scope2 : Scope
      settings: SaveName=ScopeData2
  T_fuel,T_average : Outport
  T_hot : Outport  Port=2
  wires:
  MATLAB Function/2(x_dot) -> Integrator1/1
  Integrator1/1 -> Display/1, MATLAB Function/5(x)
  m_dot -mass flow in/1 -> MATLAB Function/1(m_dot)
  Demux/2 -> Scope1/1, Mux/2  "T_average"
  T_c/1 -> MATLAB Function/4(T_c)
  From Workspace/1 -> MATLAB Function/3(constants)
  Q_rx/1 -> MATLAB Function/2(Q_rx)
  MATLAB Function/1(y) -> Demux/1
  Demux/1 -> Mux/1  "T_fuel"
  Mux/1 -> Scope2/1, T_fuel,T_average/1
  Demux/3 -> T_hot/1, Scope/1  "T_hot"

== system SpatialKineticsOffline/RX #2/Neutron Kinetics and Thermal Hydraulics1/Temperature Reactivity Feedback1 ==
  In1 : Inport
  Sum : Sum  Inputs=|+-
  reactivity feedback matrix : Gain  Gain=alpha  Multiplication=Matrix(K*u)
  reactivity reference temperature : Constant  Value=xfc0  VectorParams1D=off
  Out1 : Outport
  wires:
  reactivity reference temperature/1 -> Sum/2
  Sum/1 -> reactivity feedback matrix/1
  reactivity feedback matrix/1 -> Out1/1
  In1/1 -> Sum/1

== system SpatialKineticsOffline/RX #2/Neutron Kinetics and Thermal Hydraulics1/Temperature Reactivity Feedback2 ==
  In1 : Inport
  Sum : Sum  Inputs=|+-
  reactivity feedback matrix : Gain  Gain=alpha  Multiplication=Matrix(K*u)
  reactivity reference temperature : Constant  Value=xfc0  VectorParams1D=off
  Out1 : Outport
  wires:
  reactivity reference temperature/1 -> Sum/2
  Sum/1 -> reactivity feedback matrix/1
  reactivity feedback matrix/1 -> Out1/1
  In1/1 -> Sum/1

== system SpatialKineticsOffline/RX #2/Neutron Kinetics and Thermal Hydraulics1/Temperature Reactivity Feedback3 ==
  In1 : Inport
  Sum : Sum  Inputs=|+-
  reactivity feedback matrix : Gain  Gain=alpha  Multiplication=Matrix(K*u)
  reactivity reference temperature : Constant  Value=xfc0  VectorParams1D=off
  Out1 : Outport
  wires:
  reactivity reference temperature/1 -> Sum/2
  Sum/1 -> reactivity feedback matrix/1
  reactivity feedback matrix/1 -> Out1/1
  In1/1 -> Sum/1

== system SpatialKineticsOffline/RX #3/Neutron Kinetics and Thermal Hydraulics1/Reactor Thermal-Hydraulics Zone 1 ==
  Q_rx : Inport
  m_dot -mass flow in : Inport  Port=2
  T_c : Inport  Port=3
  Demux : Demux  Outputs=3
  Display : Display
  From Workspace : FromWorkspace  VariableName=[0,cpc,cpf,mc,mf,uh,Ar]  SampleTime=0
  Integrator1 : Integrator  InitialCondition=zone1_thermal_IO
  MATLAB Function : MATLAB Function  TreatAsAtomicUnit=on
  Mux : Mux  Inputs=2
  Scope : Scope
      settings: SaveName=ScopeData8
  Scope1 : Scope
      settings: SaveName=ScopeData9
  Scope2 : Scope
      settings: SaveName=ScopeData2
  T_fuel,T_average : Outport
  T_hot : Outport  Port=2
  wires:
  MATLAB Function/2(x_dot) -> Integrator1/1
  Integrator1/1 -> Display/1, MATLAB Function/5(x)
  m_dot -mass flow in/1 -> MATLAB Function/1(m_dot)
  Demux/2 -> Scope1/1, Mux/2  "T_average"
  T_c/1 -> MATLAB Function/4(T_c)
  From Workspace/1 -> MATLAB Function/3(constants)
  Q_rx/1 -> MATLAB Function/2(Q_rx)
  MATLAB Function/1(y) -> Demux/1
  Demux/1 -> Mux/1  "T_fuel"
  Mux/1 -> Scope2/1, T_fuel,T_average/1
  Demux/3 -> T_hot/1, Scope/1  "T_hot"

== system SpatialKineticsOffline/RX #3/Neutron Kinetics and Thermal Hydraulics1/Reactor Thermal-Hydraulics Zone 2 ==
  Q_rx : Inport
  m_dot -mass flow in : Inport  Port=2
  T_c : Inport  Port=3
  Demux : Demux  Outputs=3
  Display : Display
  From Workspace : FromWorkspace  VariableName=[0,cpc,cpf,mc,mf,uh,Ar]  SampleTime=0
  Integrator1 : Integrator  InitialCondition=zone2_thermal_IO
  MATLAB Function : MATLAB Function  TreatAsAtomicUnit=on
  Mux : Mux  Inputs=2
  Scope : Scope
      settings: SaveName=ScopeData8
  Scope1 : Scope
      settings: SaveName=ScopeData9
  Scope2 : Scope
      settings: SaveName=ScopeData2
  T_fuel,T_average : Outport
  T_hot : Outport  Port=2
  wires:
  MATLAB Function/2(x_dot) -> Integrator1/1
  Integrator1/1 -> Display/1, MATLAB Function/5(x)
  m_dot -mass flow in/1 -> MATLAB Function/1(m_dot)
  Demux/2 -> Scope1/1, Mux/2  "T_average"
  T_c/1 -> MATLAB Function/4(T_c)
  From Workspace/1 -> MATLAB Function/3(constants)
  Q_rx/1 -> MATLAB Function/2(Q_rx)
  MATLAB Function/1(y) -> Demux/1
  Demux/1 -> Mux/1  "T_fuel"
  Mux/1 -> Scope2/1, T_fuel,T_average/1
  Demux/3 -> T_hot/1, Scope/1  "T_hot"

== system SpatialKineticsOffline/RX #3/Neutron Kinetics and Thermal Hydraulics1/Reactor Thermal-Hydraulics Zone 3 ==
  Q_rx : Inport
  m_dot -mass flow in : Inport  Port=2
  T_c : Inport  Port=3
  Demux : Demux  Outputs=3
  Display : Display
  From Workspace : FromWorkspace  VariableName=[0,cpc,cpf,mc,mf,uh,Ar]  SampleTime=0
  Integrator1 : Integrator  InitialCondition=zone3_thermal_IO
  MATLAB Function : MATLAB Function  TreatAsAtomicUnit=on
  Mux : Mux  Inputs=2
  Scope : Scope
      settings: SaveName=ScopeData8
  Scope1 : Scope
      settings: SaveName=ScopeData9
  Scope2 : Scope
      settings: SaveName=ScopeData2
  T_fuel,T_average : Outport
  T_hot : Outport  Port=2
  wires:
  MATLAB Function/2(x_dot) -> Integrator1/1
  Integrator1/1 -> Display/1, MATLAB Function/5(x)
  m_dot -mass flow in/1 -> MATLAB Function/1(m_dot)
  Demux/2 -> Scope1/1, Mux/2  "T_average"
  T_c/1 -> MATLAB Function/4(T_c)
  From Workspace/1 -> MATLAB Function/3(constants)
  Q_rx/1 -> MATLAB Function/2(Q_rx)
  MATLAB Function/1(y) -> Demux/1
  Demux/1 -> Mux/1  "T_fuel"
  Mux/1 -> Scope2/1, T_fuel,T_average/1
  Demux/3 -> T_hot/1, Scope/1  "T_hot"

== system SpatialKineticsOffline/RX #3/Neutron Kinetics and Thermal Hydraulics1/Temperature Reactivity Feedback1 ==
  In1 : Inport
  Sum : Sum  Inputs=|+-
  reactivity feedback matrix : Gain  Gain=alpha  Multiplication=Matrix(K*u)
  reactivity reference temperature : Constant  Value=xfc0  VectorParams1D=off
  Out1 : Outport
  wires:
  reactivity reference temperature/1 -> Sum/2
  Sum/1 -> reactivity feedback matrix/1
  reactivity feedback matrix/1 -> Out1/1
  In1/1 -> Sum/1

== system SpatialKineticsOffline/RX #3/Neutron Kinetics and Thermal Hydraulics1/Temperature Reactivity Feedback2 ==
  In1 : Inport
  Sum : Sum  Inputs=|+-
  reactivity feedback matrix : Gain  Gain=alpha  Multiplication=Matrix(K*u)
  reactivity reference temperature : Constant  Value=xfc0  VectorParams1D=off
  Out1 : Outport
  wires:
  reactivity reference temperature/1 -> Sum/2
  Sum/1 -> reactivity feedback matrix/1
  reactivity feedback matrix/1 -> Out1/1
  In1/1 -> Sum/1

== system SpatialKineticsOffline/RX #3/Neutron Kinetics and Thermal Hydraulics1/Temperature Reactivity Feedback3 ==
  In1 : Inport
  Sum : Sum  Inputs=|+-
  reactivity feedback matrix : Gain  Gain=alpha  Multiplication=Matrix(K*u)
  reactivity reference temperature : Constant  Value=xfc0  VectorParams1D=off
  Out1 : Outport
  wires:
  reactivity reference temperature/1 -> Sum/2
  Sum/1 -> reactivity feedback matrix/1
  reactivity feedback matrix/1 -> Out1/1
  In1/1 -> Sum/1

== system SpatialKineticsOffline/RX #4/Neutron Kinetics and Thermal Hydraulics/Reactor Thermal-Hydraulics Zone 1 ==
  Q_rx : Inport
  m_dot -mass flow in : Inport  Port=2
  T_c : Inport  Port=3
  Demux : Demux  Outputs=3
  Display : Display
  From Workspace : FromWorkspace  VariableName=[0,cpc,cpf,mc,mf,uh,Ar]  SampleTime=0
  Integrator1 : Integrator  InitialCondition=zone1_thermal_IO
  MATLAB Function : MATLAB Function  TreatAsAtomicUnit=on
  Mux : Mux  Inputs=2
  Scope : Scope
      settings: SaveName=ScopeData8
  Scope1 : Scope
      settings: SaveName=ScopeData9
  Scope2 : Scope
      settings: SaveName=ScopeData2
  T_fuel,T_average : Outport
  T_hot : Outport  Port=2
  wires:
  MATLAB Function/2(x_dot) -> Integrator1/1
  Integrator1/1 -> Display/1, MATLAB Function/5(x)
  m_dot -mass flow in/1 -> MATLAB Function/1(m_dot)
  Demux/2 -> Scope1/1, Mux/2  "T_average"
  T_c/1 -> MATLAB Function/4(T_c)
  From Workspace/1 -> MATLAB Function/3(constants)
  Q_rx/1 -> MATLAB Function/2(Q_rx)
  MATLAB Function/1(y) -> Demux/1
  Demux/1 -> Mux/1  "T_fuel"
  Mux/1 -> Scope2/1, T_fuel,T_average/1
  Demux/3 -> T_hot/1, Scope/1  "T_hot"

== system SpatialKineticsOffline/RX #4/Neutron Kinetics and Thermal Hydraulics/Reactor Thermal-Hydraulics Zone 2 ==
  Q_rx : Inport
  m_dot -mass flow in : Inport  Port=2
  T_c : Inport  Port=3
  Demux : Demux  Outputs=3
  Display : Display
  From Workspace : FromWorkspace  VariableName=[0,cpc,cpf,mc,mf,uh,Ar]  SampleTime=0
  Integrator1 : Integrator  InitialCondition=zone2_thermal_IO
  MATLAB Function : MATLAB Function  TreatAsAtomicUnit=on
  Mux : Mux  Inputs=2
  Scope : Scope
      settings: SaveName=ScopeData8
  Scope1 : Scope
      settings: SaveName=ScopeData9
  Scope2 : Scope
      settings: SaveName=ScopeData2
  T_fuel,T_average : Outport
  T_hot : Outport  Port=2
  wires:
  MATLAB Function/2(x_dot) -> Integrator1/1
  Integrator1/1 -> Display/1, MATLAB Function/5(x)
  m_dot -mass flow in/1 -> MATLAB Function/1(m_dot)
  Demux/2 -> Scope1/1, Mux/2  "T_average"
  T_c/1 -> MATLAB Function/4(T_c)
  From Workspace/1 -> MATLAB Function/3(constants)
  Q_rx/1 -> MATLAB Function/2(Q_rx)
  MATLAB Function/1(y) -> Demux/1
  Demux/1 -> Mux/1  "T_fuel"
  Mux/1 -> Scope2/1, T_fuel,T_average/1
  Demux/3 -> T_hot/1, Scope/1  "T_hot"

== system SpatialKineticsOffline/RX #4/Neutron Kinetics and Thermal Hydraulics/Reactor Thermal-Hydraulics Zone 3 ==
  Q_rx : Inport
  m_dot -mass flow in : Inport  Port=2
  T_c : Inport  Port=3
  Demux : Demux  Outputs=3
  Display : Display
  From Workspace : FromWorkspace  VariableName=[0,cpc,cpf,mc,mf,uh,Ar]  SampleTime=0
  Integrator1 : Integrator  InitialCondition=zone3_thermal_IO
  MATLAB Function : MATLAB Function  TreatAsAtomicUnit=on
  Mux : Mux  Inputs=2
  Scope : Scope
      settings: SaveName=ScopeData8
  Scope1 : Scope
      settings: SaveName=ScopeData9
  Scope2 : Scope
      settings: SaveName=ScopeData2
  T_fuel,T_average : Outport
  T_hot : Outport  Port=2
  wires:
  MATLAB Function/2(x_dot) -> Integrator1/1
  Integrator1/1 -> Display/1, MATLAB Function/5(x)
  m_dot -mass flow in/1 -> MATLAB Function/1(m_dot)
  Demux/2 -> Scope1/1, Mux/2  "T_average"
  T_c/1 -> MATLAB Function/4(T_c)
  From Workspace/1 -> MATLAB Function/3(constants)
  Q_rx/1 -> MATLAB Function/2(Q_rx)
  MATLAB Function/1(y) -> Demux/1
  Demux/1 -> Mux/1  "T_fuel"
  Mux/1 -> Scope2/1, T_fuel,T_average/1
  Demux/3 -> T_hot/1, Scope/1  "T_hot"

== system SpatialKineticsOffline/RX #4/Neutron Kinetics and Thermal Hydraulics/Temperature Reactivity Feedback1 ==
  In1 : Inport
  Sum : Sum  Inputs=|+-
  reactivity feedback matrix : Gain  Gain=alpha  Multiplication=Matrix(K*u)
  reactivity reference temperature : Constant  Value=xfc0  VectorParams1D=off
  Out1 : Outport
  wires:
  reactivity reference temperature/1 -> Sum/2
  Sum/1 -> reactivity feedback matrix/1
  reactivity feedback matrix/1 -> Out1/1
  In1/1 -> Sum/1
